simulink model "Pressure_Drop_changeD_1"  (Simulink 7.6)
settings: Solver=ode45  StartTime=0.0  StopTime=10.0  RelTol=1e-3
libraries: carnot x2
settings Model: Creator=drhf  LastModifiedBy=drhf

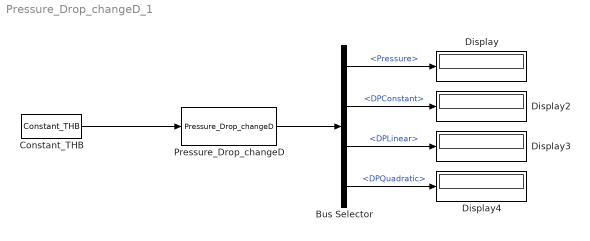
== system Pressure_Drop_changeD_1 ==
  Bus Selector : BusSelector  OutputSignals=Pressure,DPConstant,DPLinear,DPQuadratic
  Constant_THB : carnot/Source/Simple/Constant_THB  SystemSampleTime=-1  t=40  mdot=100/3600  p=1e5  mID=Full Pressure Drop with Static Height  fluid=water  mix=0  dia=1  hgt=0
  Display{,2..4} (4 alike) : Display
  Pressure_Drop_changeD : carnot/Basic/Pressure_Drop/Pressure_Drop_changeD  SystemSampleTime=-1  dia=0.02  height=1
  wires:
  Constant_THB/1 -> Pressure_Drop_changeD/1
  Pressure_Drop_changeD/1 -> Bus Selector/1
  Bus Selector/1 -> Display/1  "<Pressure>"
  Bus Selector/2 -> Display2/1  "<DPConstant>"
  Bus Selector/3 -> Display3/1  "<DPLinear>"
  Bus Selector/4 -> Display4/1  "<DPQuadratic>"
